simulink model "stdMRS"  (R2014a)
settings: Solver=ode45  StartTime=0.0  StopTime=20  RelTol=1e-3
settings Model: Creator=cocoa  LastModifiedBy=cocoa

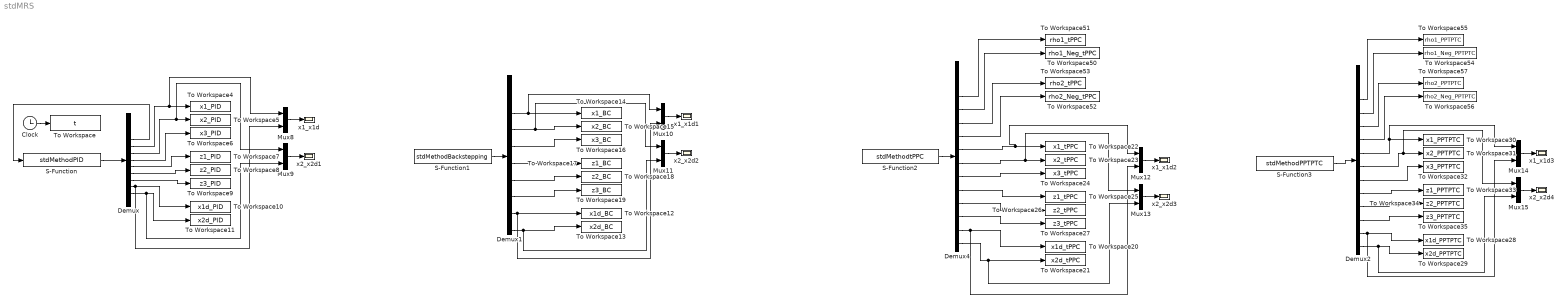
== system stdMRS ==
  Clock : Clock
  Demux : Demux  Outputs=11
  Demux1 : Demux  Outputs=10
  Demux2 : Demux  Outputs=14
  Demux4 : Demux  Outputs=14
  Mux{8..15} (8 alike) : Mux  Inputs=2
  S-Function : S-Function  FunctionName=stdMethodPID  EnableBusSupport=off
  S-Function1 : S-Function  FunctionName=stdMethodBackstepping  EnableBusSupport=off
  S-Function2 : S-Function  FunctionName=stdMethodtPPC  EnableBusSupport=off
  S-Function3 : S-Function  FunctionName=stdMethodPPTPTC  EnableBusSupport=off
  To Workspace : ToWorkspace  VariableName=t  SaveFormat=Timeseries  SampleTime=-1
  To Workspace10 : ToWorkspace  VariableName=x1d_PID  SaveFormat=Timeseries  SampleTime=-1
  To Workspace11 : ToWorkspace  VariableName=x2d_PID  SaveFormat=Timeseries  SampleTime=-1
  To Workspace12 : ToWorkspace  VariableName=x1d_BC  SaveFormat=Timeseries  SampleTime=-1
  To Workspace13 : ToWorkspace  VariableName=x2d_BC  SaveFormat=Timeseries  SampleTime=-1
  To Workspace14 : ToWorkspace  VariableName=x1_BC  SaveFormat=Timeseries  SampleTime=-1
  To Workspace15 : ToWorkspace  VariableName=x2_BC  SaveFormat=Timeseries  SampleTime=-1
  To Workspace16 : ToWorkspace  VariableName=x3_BC  SaveFormat=Timeseries  SampleTime=-1
  To Workspace17 : ToWorkspace  VariableName=z1_BC  SaveFormat=Timeseries  SampleTime=-1
  To Workspace18 : ToWorkspace  VariableName=z2_BC  SaveFormat=Timeseries  SampleTime=-1
  To Workspace19 : ToWorkspace  VariableName=z3_BC  SaveFormat=Timeseries  SampleTime=-1
  To Workspace20 : ToWorkspace  VariableName=x1d_tPPC  SaveFormat=Timeseries  SampleTime=-1
  To Workspace21 : ToWorkspace  VariableName=x2d_tPPC  SaveFormat=Timeseries  SampleTime=-1
  To Workspace22 : ToWorkspace  VariableName=x1_tPPC  SaveFormat=Timeseries  SampleTime=-1
  To Workspace23 : ToWorkspace  VariableName=x2_tPPC  SaveFormat=Timeseries  SampleTime=-1
  To Workspace24 : ToWorkspace  VariableName=x3_tPPC  SaveFormat=Timeseries  SampleTime=-1
  To Workspace25 : ToWorkspace  VariableName=z1_tPPC  SaveFormat=Timeseries  SampleTime=-1
  To Workspace26 : ToWorkspace  VariableName=z2_tPPC  SaveFormat=Timeseries  SampleTime=-1
  To Workspace27 : ToWorkspace  VariableName=z3_tPPC  SaveFormat=Timeseries  SampleTime=-1
  To Workspace28 : ToWorkspace  VariableName=x1d_PPTPTC  SaveFormat=Timeseries  SampleTime=-1
  To Workspace29 : ToWorkspace  VariableName=x2d_PPTPTC  SaveFormat=Timeseries  SampleTime=-1
  To Workspace30 : ToWorkspace  VariableName=x1_PPTPTC  SaveFormat=Timeseries  SampleTime=-1
  To Workspace31 : ToWorkspace  VariableName=x2_PPTPTC  SaveFormat=Timeseries  SampleTime=-1
  To Workspace32 : ToWorkspace  VariableName=x3_PPTPTC  SaveFormat=Timeseries  SampleTime=-1
  To Workspace33 : ToWorkspace  VariableName=z1_PPTPTC  SaveFormat=Timeseries  SampleTime=-1
  To Workspace34 : ToWorkspace  VariableName=z2_PPTPTC  SaveFormat=Timeseries  SampleTime=-1
  To Workspace35 : ToWorkspace  VariableName=z3_PPTPTC  SaveFormat=Timeseries  SampleTime=-1
  To Workspace4 : ToWorkspace  VariableName=x1_PID  SaveFormat=Timeseries  SampleTime=-1
  To Workspace5 : ToWorkspace  VariableName=x2_PID  SaveFormat=Timeseries  SampleTime=-1
  To Workspace50 : ToWorkspace  VariableName=rho1_Neg_tPPC  SaveFormat=Timeseries  SampleTime=-1
  To Workspace51 : ToWorkspace  VariableName=rho1_tPPC  SaveFormat=Timeseries  SampleTime=-1
  To Workspace52 : ToWorkspace  VariableName=rho2_Neg_tPPC  SaveFormat=Timeseries  SampleTime=-1
  To Workspace53 : ToWorkspace  VariableName=rho2_tPPC  SaveFormat=Timeseries  SampleTime=-1
  To Workspace54 : ToWorkspace  VariableName=rho1_Neg_PPTPTC  SaveFormat=Timeseries  SampleTime=-1
  To Workspace55 : ToWorkspace  VariableName=rho1_PPTPTC  SaveFormat=Timeseries  SampleTime=-1
  To Workspace56 : ToWorkspace  VariableName=rho2_Neg_PPTPTC  SaveFormat=Timeseries  SampleTime=-1
  To Workspace57 : ToWorkspace  VariableName=rho2_PPTPTC  SaveFormat=Timeseries  SampleTime=-1
  To Workspace6 : ToWorkspace  VariableName=x3_PID  SaveFormat=Timeseries  SampleTime=-1
  To Workspace7 : ToWorkspace  VariableName=z1_PID  SaveFormat=Timeseries  SampleTime=-1
  To Workspace8 : ToWorkspace  VariableName=z2_PID  SaveFormat=Timeseries  SampleTime=-1
  To Workspace9 : ToWorkspace  VariableName=z3_PID  SaveFormat=Timeseries  SampleTime=-1
  x1_x1d{,1..3} (4 alike) : Scope
      x1_x1d settings: SaveName=ScopeData58
      x1_x1d2 settings: SaveName=ScopeData2
      x1_x1d3 settings: SaveName=ScopeData4
  x2_x2d{1..4} (4 alike) : Scope
      x2_x2d1 settings: SaveName=ScopeData59
      x2_x2d3 settings: SaveName=ScopeData3
      x2_x2d4 settings: SaveName=ScopeData32
  wires:
  S-Function/1 -> Demux/1
  Clock/1 -> To Workspace/1
  Demux/3 -> S-Function/1
  S-Function1/1 -> Demux1/1
  S-Function2/1 -> Demux4/1
  S-Function3/1 -> Demux2/1
  Demux1/10 -> Mux11/2, To Workspace13/1
  Mux8/1 -> x1_x1d/1
  Mux9/1 -> x2_x2d1/1
  Demux/5 -> To Workspace5/1, Mux9/1
  Demux/6 -> To Workspace6/1
  Demux/7 -> To Workspace7/1
  Demux/8 -> To Workspace8/1
  Demux/9 -> To Workspace9/1
  Demux/10 -> Mux8/2, To Workspace10/1
  Demux/11 -> Mux9/2, To Workspace11/1
  Demux/4 -> Mux8/1, To Workspace4/1
  Mux10/1 -> x1_x1d1/1
  Mux11/1 -> x2_x2d2/1
  Demux1/3 -> Mux10/1, To Workspace14/1
  Demux1/4 -> Mux11/1, To Workspace15/1
  Demux1/5 -> To Workspace16/1
  Demux1/6 -> To Workspace17/1
  Demux1/7 -> To Workspace18/1
  Demux1/8 -> To Workspace19/1
  Demux1/9 -> Mux10/2, To Workspace12/1
  Mux12/1 -> x1_x1d2/1
  Mux13/1 -> x2_x2d3/1
  Demux4/7 -> Mux12/1, To Workspace22/1
  Demux4/8 -> Mux13/1, To Workspace23/1
  Demux4/9 -> To Workspace24/1
  Demux4/10 -> To Workspace25/1
  Demux4/11 -> To Workspace26/1
  Demux4/12 -> To Workspace27/1
  Demux4/13 -> Mux12/2, To Workspace20/1
  Demux4/14 -> Mux13/2, To Workspace21/1
  Mux14/1 -> x1_x1d3/1
  Mux15/1 -> x2_x2d4/1
  Demux2/7 -> Mux14/1, To Workspace30/1
  Demux2/8 -> Mux15/1, To Workspace31/1
  Demux2/9 -> To Workspace32/1
  Demux2/10 -> To Workspace33/1
  Demux2/11 -> To Workspace34/1
  Demux2/12 -> To Workspace35/1
  Demux2/13 -> Mux14/2, To Workspace28/1
  Demux2/14 -> Mux15/2, To Workspace29/1
  Demux4/3 -> To Workspace51/1
  Demux4/4 -> To Workspace50/1
  Demux4/5 -> To Workspace53/1
  Demux4/6 -> To Workspace52/1
  Demux2/3 -> To Workspace55/1
  Demux2/4 -> To Workspace54/1
  Demux2/5 -> To Workspace57/1
  Demux2/6 -> To Workspace56/1
